simulink model "Odwrotny_model_Odniesienia"  (R2019b)
settings: Solver=VariableStepAuto  StartTime=0.0  StopTime=100  RelTol=1e-3
values from neighbouring files (symbols this model uses):
  A = [0 -2;1 2]    [Skrypt.m]
  B = [0;1]    [Skrypt.m]
  C = [4 0]    [Skrypt.m]
  D = 0    [Skrypt.m]
  Kx = -place(A,B,s)    [Skrypt.m]
  Lo = acker(A',C',s2)    [Skrypt.m]
settings Model: Creator=szymo  LastModifiedBy=szymo

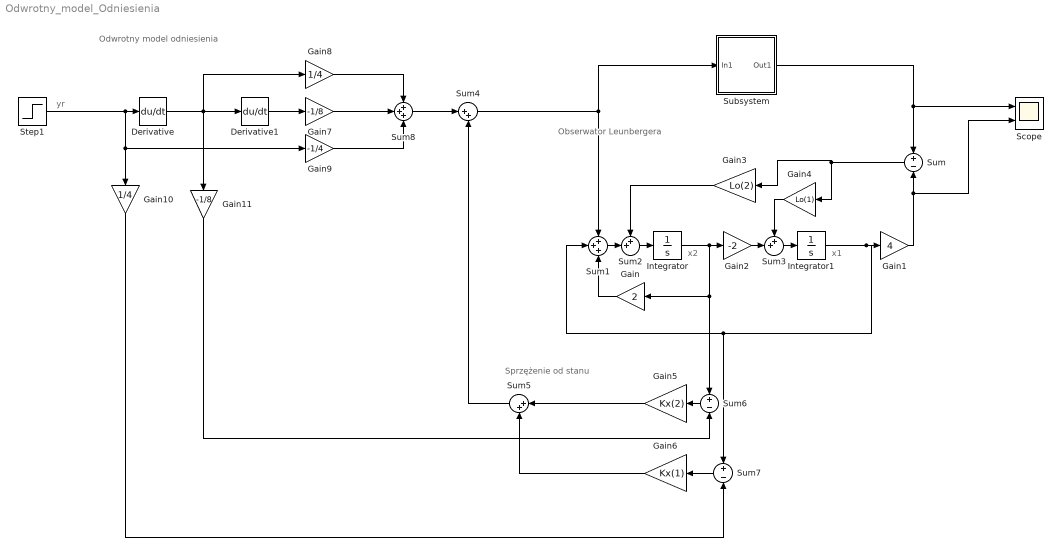
== system Odwrotny_model_Odniesienia ==
  note: Odwrotny model odniesienia
  note: yr
  note: Sprzężenie od stanu
  note: x1
  note: Obserwator Leunbergera
  note: x2
  Derivative : Derivative
  Derivative1 : Derivative
  Gain : Gain  Gain=2
  Gain1 : Gain  Gain=4
  Gain10 : Gain  Gain=1/4
  Gain11 : Gain  Gain=-1/8
  Gain2 : Gain  Gain=-2
  Gain3 : Gain  Gain=Lo(2)
  Gain4 : Gain  Gain=Lo(1)
  Gain5 : Gain  Gain=Kx(2)
  Gain6 : Gain  Gain=Kx(1)
  Gain7 : Gain  Gain=-1/8
  Gain8 : Gain  Gain=1/4
  Gain9 : Gain  Gain=-1/4
  Integrator : Integrator
  Integrator1 : Integrator
  Scope : Scope  NumInputPorts=2
  Step1 : Step  Time=0  After=28  SampleTime=0
  Subsystem : Subsystem
  Sum : Sum  Inputs=+-
  Sum1 : Sum  Inputs=+++
  Sum2 : Sum  Inputs=++|
  Sum3 : Sum  Inputs=++|
  Sum4 : Sum  Inputs=|++
  Sum5 : Sum  Inputs=|++
  Sum6 : Sum  Inputs=+-
  Sum7 : Sum  Inputs=+-
  Sum8 : Sum  Inputs=+++
  wires:
  Subsystem/1(Out1) -> Sum/1, Scope/1
  Integrator/1 -> Gain2/1, Sum6/1, Gain/1
  Gain/1 -> Sum1/3
  Integrator1/1 -> Sum1/2, Sum7/1, Gain1/1
  Sum1/1 -> Sum2/2
  Sum2/1 -> Integrator/1
  Gain3/1 -> Sum2/1
  Sum/1 -> Gain4/1, Gain3/1
  Gain2/1 -> Sum3/2
  Sum3/1 -> Integrator1/1
  Gain4/1 -> Sum3/1
  Gain1/1 -> Scope/2, Sum/2
  Sum4/1 -> Sum1/1, Subsystem/1(In1)
  Gain6/1 -> Sum5/2
  Gain5/1 -> Sum5/1
  Sum6/1 -> Gain5/1
  Sum7/1 -> Gain6/1
  Gain7/1 -> Sum8/2
  Sum5/1 -> Sum4/2
  Derivative/1 -> Gain11/1, Gain8/1, Derivative1/1
  Step1/1 -> Gain10/1, Gain9/1, Derivative/1
  Derivative1/1 -> Gain7/1
  Gain8/1 -> Sum8/1
  Gain9/1 -> Sum8/3
  Gain10/1 -> Sum7/2
  Gain11/1 -> Sum6/2
  Sum8/1 -> Sum4/1

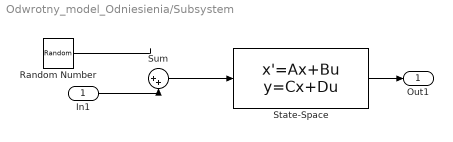
== system Odwrotny_model_Odniesienia/Subsystem ==
  In1 : Inport
  Random Number : RandomNumber  Mean=0.5  SampleTime=0.1
  State-Space : StateSpace  A=A  B=B  C=C  D=D  InitialCondition=0
  Sum : Sum  Inputs=|++
  Out1 : Outport
  wires:
  In1/1 -> Sum/2
  Sum/1 -> State-Space/1
  State-Space/1 -> Out1/1
  Random Number/1 -> ?
